simulink model "Pitch_Rate_Damper"  (R2024b)
settings: Solver=VariableStepAuto  StartTime=0.0  StopTime=5  RelTol=1e-3
undefined symbols (not defined in the file): Kp_1
libraries: slpidlib x1
settings Model: Creator=GH-X-ST  LastModifiedBy=GH-X-ST

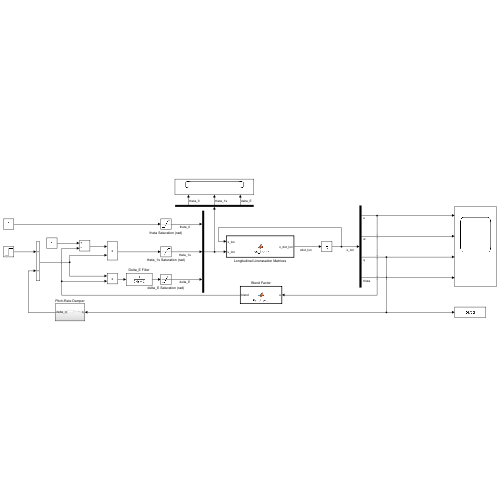
[thumbnail: Simulink's stored preview of the top-level diagram]
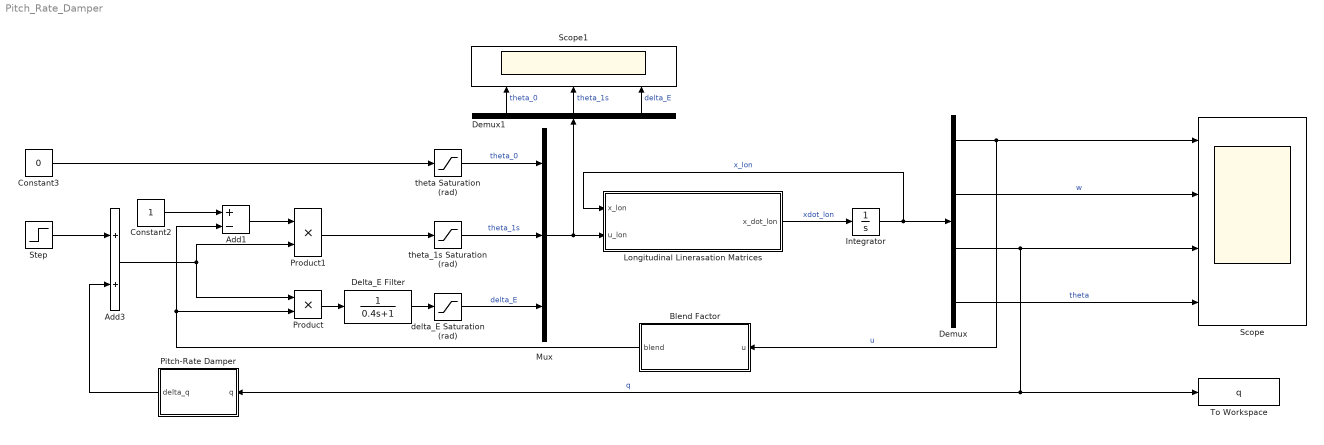
== system Pitch_Rate_Damper ==
  Add1 : Sum  Inputs=+-
  Add3 : Sum
  Blend Factor : MATLAB Function  TreatAsAtomicUnit=on
  Constant2 : Constant
  Constant3 : Constant  Value=0
  Delta_E Filter : TransferFcn  Denominator=[0.4 1]
  Demux : Demux
  Demux1 : Demux  Outputs=3
  Integrator : Integrator  InitialCondition=[0;0;0;0]
  Longitudinal Linerasation Matrices : MATLAB Function  TreatAsAtomicUnit=on
  Mux : Mux  Inputs=3
  Pitch-Rate Damper : Subsystem
  Product : Product
  Product1 : Product
  Scope : Scope  NumInputPorts=4
  Scope1 : Scope  NumInputPorts=3
  Step : Step  After=0.005  SampleTime=0
  To Workspace : ToWorkspace  VariableName=q  SaveFormat=Timeseries  SampleTime=-1
  delta_E Saturation (rad) : Saturate  UpperLimit=deg2rad(11)  LowerLimit=deg2rad(-11)
  theta Saturation (rad) : Saturate  UpperLimit=deg2rad(20)  LowerLimit=0
  theta_1s Saturation (rad) : Saturate  UpperLimit=deg2rad(6)  LowerLimit=deg2rad(-6)
  wires:
  Longitudinal Linerasation Matrices/1(x_dot_lon) -> Integrator/1  "xdot_lon"
  Integrator/1 -> Longitudinal Linerasation Matrices/1(x_lon), Demux/1  "x_lon"
  Demux/1 -> Blend Factor/1(u), Scope/1  "u"
  Demux/2 -> Scope/2  "w"
  Demux/3 -> Scope/3, Pitch-Rate Damper/1(q), To Workspace/1  "q"
  Demux/4 -> Scope/4  "theta"
  theta Saturation (rad)/1 -> Mux/1  "theta_0"
  theta_1s Saturation (rad)/1 -> Mux/2  "theta_1s"
  delta_E Saturation (rad)/1 -> Mux/3  "delta_E"
  Blend Factor/1(blend) -> Add1/2, Product/2
  Add3/1 -> Product1/2, Product/1
  Constant2/1 -> Add1/1
  Add1/1 -> Product1/1
  Mux/1 -> Demux1/1, Longitudinal Linerasation Matrices/2(u_lon)
  Demux1/3 -> Scope1/3  "delta_E"
  Demux1/2 -> Scope1/2  "theta_1s"
  Demux1/1 -> Scope1/1  "theta_0"
  Constant3/1 -> theta Saturation (rad)/1
  Product1/1 -> theta_1s Saturation (rad)/1
  Product/1 -> Delta_E Filter/1
  Delta_E Filter/1 -> delta_E Saturation (rad)/1
  Pitch-Rate Damper/1(delta_q) -> Add3/2
  Step/1 -> Add3/1

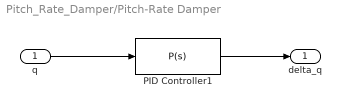
== system Pitch_Rate_Damper/Pitch-Rate Damper ==
  q : Inport
  PID Controller1 : slpidlib/PID Controller  Controller=P  Form=Parallel  TimeDomain=Continuous-time  UseExternalTs=off  SampleTime=-1  IntegratorMethod=Forward Euler  FilterMethod=Forward Euler  ControllerParametersSource=internal  P=Kp_1  I=0.005  UseKiTs=off  D=0.005  UseExternalDerivativeSource=on  N=100  UseFilter=on  TunerSelectOption=Transfer Function Based (PID Tuner App)  InitialConditionSource=internal  InitialConditionForIntegrator=0  InitialConditionForFilter=0  DifferentiatorICPrevScaledInput=0  ExternalReset=none  TrackingMode=off  Kt=1  LimitOutput=on  SatLimitsSource=internal  UpperSaturationLimit=1  LowerSaturationLimit=-1  LinearizeAsGain=on  AntiWindupMode=none  Kb=1  LimitIntegrator=off  UpperIntegratorSaturationLimit=inf  LowerIntegratorSaturationLimit=-inf  POutMin=[]  POutMax=[]  IOutMin=[]  IOutMax=[]  DOutMin=[]  DOutMax=[]  NOutMin=[]  NOutMax=[]  SumOutMin=[]  SumOutMax=[]  SaturationOutMin=[]  SaturationOutMax=[]  PParamMin=[]  PParamMax=[]  IParamMin=[]  IParamMax=[]  DParamMin=[]  DParamMax=[]  NParamMin=[]  NParamMax=[]  KbParamMin=[]  KbParamMax=[]  KtParamMin=[]  KtParamMax=[]  KbOutMin=[]  KbOutMax=[]  KtOutMin=[]  KtOutMax=[]  IntegratorOutMin=[]  IntegratorOutMax=[]  FilterOutMin=[]  FilterOutMax=[]  SumI1OutMin=[]  SumI1OutMax=[]  SumI2OutMin=[]  SumI2OutMax=[]  SumI3OutMin=[]  SumI3OutMax=[]  SumI4OutMin=[]  SumI4OutMax=[]  SumDOutMin=[]  SumDOutMax=[]  DifferentiatorOutMin=[]  DifferentiatorOutMax=[]  FilterDiffOutCoefMin=[]  FilterDiffOutCoefMax=[]  ReciprocalOutMin=[]  ReciprocalOutMax=[]  SumDenOutMin=[]  SumDenOutMax=[]  SumNumOutMin=[]  SumNumOutMax=[]  DivideOutMin=[]  DivideOutMax=[]  UdiffTsProdOutMin=[]  UdiffTsProdOutMax=[]  NTsProdOutMin=[]  NTsProdOutMax=[]  UintegralTsProdOutMin=[]  UintegralTsProdOutMax=[]  UngainTsProdOutMin=[]  UngainTsProdOutMax=[]  ClampingZeroOutDataTypeStr=Inherit: Inherit via back propagation  ClampingZeroOutMin=[]  ClampingZeroOutMax=[]  FilterDenConstantOutDataTypeStr=Inherit: Inherit via back propagation  FilterDenConstantOutMin=[]  FilterDenConstantOutMax=[]  PCopyOutDataTypeStr=Inherit: Inherit via back propagation  PCopyOutMin=[]  PCopyOutMax=[]  NCopyOutDataTypeStr=Inherit: Inherit via back propagation  NCopyOutMin=[]  NCopyOutMax=[]  IntegratorContinuousStateAttributes=''  IntegratorStateMustResolveToSignalObject=off  IntegratorRTWStateStorageClass=Auto  FilterContinuousStateAttributes=''  FilterStateMustResolveToSignalObject=off  FilterRTWStateStorageClass=Auto  ParallelPVariant=InternalParameters  IdealPVariant=Disabled  IVariant=Disabled  DVariant=Disabled  IntegratorVariant=Disabled  SatVariant=Enabled  AWVariant=Disabled  PCopyVariant=Disabled  TRVariant=Disabled  FdbkBlocksVariant=Forward  IdealPFdbkVariant=Disabled  SatFdbkVariant=Disabled  DerivativeFilterVariant=Disabled  NVariant=Passthrough  NCopyVariant=Disabled_SignalSpec  FilterICVariant=Disabled  IntegratorICVariant=Disabled  ExternalResetVariant=Disabled  TRSumVariant=Passthrough  SumFdbkVariant=Disabled  SumVariant=Passthrough_P  TsampFilterVariant=InternalTs  TsampNgainVariant=Passthrough  TsampIntegralVariant=Disabled_SignalSpec  ExternalSaturationOutDataTypeStr=Inherit: Same as second input  DerivativeSourceVariant=Disabled  PreIntVariant=InternalPreInt
  delta_q : Outport
  wires:
  PID Controller1/1 -> delta_q/1
  q/1 -> PID Controller1/1

== matlab function Pitch_Rate_Damper/Longitudinal Linerasation Matrices ==
  data: x_lon input; u_lon input; x_dot_lon output
function x_dot_lon = Lon_linear(x_lon, u_lon)
% Author:
%   Hanchen Li (hl3422@ic.ac.uk)
%
% Inputs:
%   x_lon     - [u, w, q, theta]
%   u         - Forward velocity (m/s)
%   w         - Vertical velocity (m/s)
%   q         - Pitch rate (rad/s)
%   theta     - Euler pitch angle (rad)
%
%   u_lon     - [theta_0, theta_1s, delta_E]
%   theta_0   - Average rotor collective (rad)
%   theta_1s  - Longitudinal cyclic (rad)
%   delta_E   - Elevator deflection (rad)
%
% Outputs:
%   x_dot

A_lon = ...
[0.00797773730409901	0.0742775144324526	-1.21387619054530	-9.79666335749863;
-0.300981219236718	-1.37899711980971	10.9535968552343	-0.454094238238056;
0.0867879507802988	0.0518221856357636	-1.66200207187276	0;
0	0	0.999987703616044	0];

B_lon = ...
[10.6236577255089	-7.56754553412536	0.00130717492913268;
-223.536674937179	-16.2402084532332	-0.180124033315465;
-2.09157792284219	-17.4158153969991	-0.0756279848803381;
0	0	0];

%% 3 Output
x_dot_lon = A_lon * x_lon + B_lon * u_lon;

end

== matlab function Pitch_Rate_Damper/Blend Factor ==
  data: blend output; u input
function blend = Blend_pitch(u)
% Author:
%   Hanchen Li (hl3422@ic.ac.uk)
%
% Inputs:
%   u         - Forward velocity (m/s)
%
% Outputs:
%   blend     - blend factor

%% 1 Decide blend factor

if abs(u) < 1e-4

    blend = 0;

elseif abs(u) < 90.3

    blend = u / (90.3 / 0.8);

else

    blend = 0.8;

end

end
